simulink model "EZQStateCtrl"  (R2018b)
settings: Solver=FixedStepDiscrete  StartTime=0.0  StopTime=10.0  FixedStep=0.01  RelTol=1e-3
libraries: StateCtrlLib x1
settings Model: Creator=sn2xws  LastModifiedBy=sn2xws
settings DataIOCC: SaveFormat=StructureWithTime
settings OptimizationCC: DefaultParameterBehavior=Inlined  EnhancedBackFolding=on  PassReuseOutputArgsAs=Individual arguments  ZeroExternalMemoryAtStartup=off  ZeroInternalMemoryAtStartup=off  OptimizeBlockOrder=speed  DifferentSizesBufferReuse=on  OptimizationCustomize=off
settings DebuggingCC: ParameterTunabilityLossMsg=error
settings ModelReferenceCC: ModelReferenceNumInstancesAllowed=Single
settings SFSimCC: MATLABDynamicMemAlloc=off
settings RTWCC: SystemTargetFile=autosar.tlc  GenCodeOnly=on  TemplateMakefile=ert_default_tmf  Description=AUTOSAR  GenerateReport=on  IncludeHyperlinkInReport=on  LaunchReport=on  GenerateTraceInfo=on  GenerateTraceReport=on  GenerateTraceReportSl=on  GenerateTraceReportSf=on  GenerateTraceReportEml=on
settings CodeAppCC: ForceParamTrailComments=on  IgnoreCustomStorageClasses=off  OperatorAnnotations=on  SimulinkDataObjDesc=on  SFDataObjDesc=on  InsertBlockDesc=on
settings STFCustomTargetCC: TargetLangStandard=C99 (ISO)  MultiwordLength=256  ParMdlRefBuildCompliant=on  CompOptLevelCompliant=on  IncludeMdlTerminateFcn=off  CombineOutputUpdateFcns=on  SuppressErrorStatus=on  ERTCustomFileBanners=on  SupportNonFinite=off  SupportComplex=off  SupportContinuousTime=off  SupportNonInlinedSFcns=off  RemoveResetFunc=on  MATLABClassNameForMDSCustomization=Simulink.SoftwareTarget.ERTCustomization  AutosarCompliant=on  UseToolchainInfoCompliant=on  LookupTableObjectStructAxisOrder=2,1,3,4,...  LUTObjectStructOrderEvenSpacing=Size,Table,Breakpoints  SystemTargetFile=autosar.tlc
settings ERTTargetCC: TargetLangStandard=C99 (ISO)  ConcurrentExecutionCompliant=off  IncludeMdlTerminateFcn=off  SuppressErrorStatus=on  SupportNonFinite=off  SupportComplex=off  ModelStepFunctionPrototypeControlCompliant=off  CPPClassGenCompliant=off  AutosarCompliant=on  LookupTableObjectStructAxisOrder=2,1,3,4,...  LUTObjectStructOrderEvenSpacing=Size,Table,Breakpoints  InlinedParameterPlacement=NonHierarchical  ERTCustomFileTemplate=example_file_process.tlc

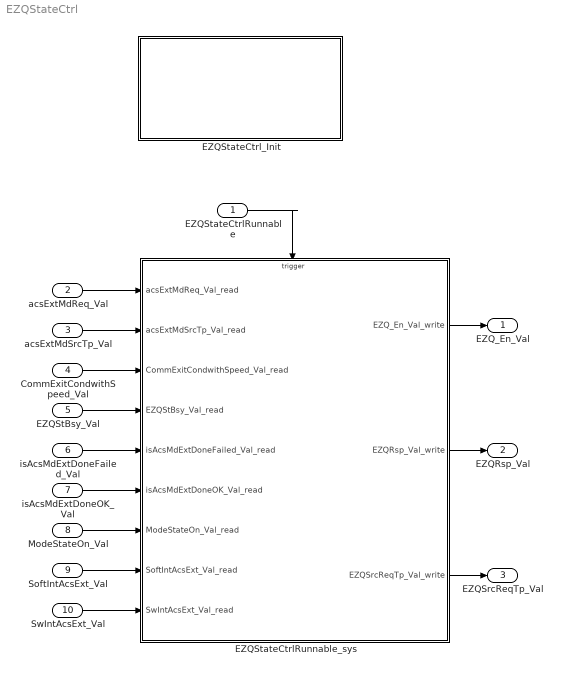
== system EZQStateCtrl ==
  EZQStateCtrlRunnable : Inport  SampleTime=0.01  OutputFunctionCall=on
  acsExtMdReq_Val : Inport  Port=2  OutDataTypeStr=boolean  PortDimensions=1
  acsExtMdSrcTp_Val : Inport  Port=3  OutDataTypeStr=Enum: SrcReqTp1  PortDimensions=1
  CommExitCondwithSpeed_Val : Inport  Port=4  OutDataTypeStr=boolean  PortDimensions=1
  EZQStBsy_Val : Inport  Port=5  OutDataTypeStr=boolean  PortDimensions=1
  isAcsMdExtDoneFailed_Val : Inport  Port=6  OutDataTypeStr=boolean  PortDimensions=1
  isAcsMdExtDoneOK_Val : Inport  Port=7  OutDataTypeStr=boolean  PortDimensions=1
  ModeStateOn_Val : Inport  Port=8  OutDataTypeStr=boolean  PortDimensions=1
  SoftIntAcsExt_Val : Inport  Port=9  OutDataTypeStr=IntEnable  PortDimensions=1
  SwIntAcsExt_Val : Inport  Port=10  OutDataTypeStr=IntEnable  PortDimensions=1
  EZQStateCtrlRunnable_sys : Subsystem
  EZQStateCtrl_Init : Subsystem
  EZQ_En_Val : Outport  OutDataTypeStr=boolean  PortDimensions=1
  EZQRsp_Val : Outport  Port=2  OutDataTypeStr=Enum: MdRspLocal1  PortDimensions=1
  EZQSrcReqTp_Val : Outport  Port=3  OutDataTypeStr=Enum: SrcReqTp1  PortDimensions=1
  wires:
  acsExtMdReq_Val/1 -> EZQStateCtrlRunnable_sys/1(acsExtMdReq_Val_read)
  acsExtMdSrcTp_Val/1 -> EZQStateCtrlRunnable_sys/2(acsExtMdSrcTp_Val_read)
  CommExitCondwithSpeed_Val/1 -> EZQStateCtrlRunnable_sys/3(CommExitCondwithSpeed_Val_read)
  EZQStBsy_Val/1 -> EZQStateCtrlRunnable_sys/4(EZQStBsy_Val_read)
  isAcsMdExtDoneFailed_Val/1 -> EZQStateCtrlRunnable_sys/5(isAcsMdExtDoneFailed_Val_read)
  isAcsMdExtDoneOK_Val/1 -> EZQStateCtrlRunnable_sys/6(isAcsMdExtDoneOK_Val_read)
  ModeStateOn_Val/1 -> EZQStateCtrlRunnable_sys/7(ModeStateOn_Val_read)
  SoftIntAcsExt_Val/1 -> EZQStateCtrlRunnable_sys/8(SoftIntAcsExt_Val_read)
  SwIntAcsExt_Val/1 -> EZQStateCtrlRunnable_sys/9(SwIntAcsExt_Val_read)
  EZQStateCtrlRunnable_sys/1(EZQ_En_Val_write) -> EZQ_En_Val/1
  EZQStateCtrlRunnable_sys/2(EZQRsp_Val_write) -> EZQRsp_Val/1
  EZQStateCtrlRunnable_sys/3(EZQSrcReqTp_Val_write) -> EZQSrcReqTp_Val/1
  EZQStateCtrlRunnable/1 -> EZQStateCtrlRunnable_sys/Trigger

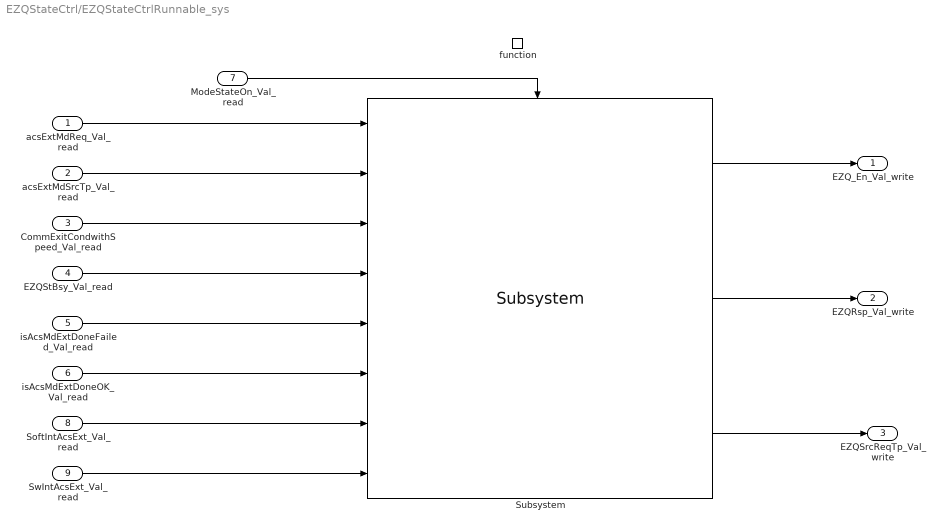
== system EZQStateCtrl/EZQStateCtrlRunnable_sys ==
  acsExtMdReq_Val_read : Inport
  acsExtMdSrcTp_Val_read : Inport  Port=2
  CommExitCondwithSpeed_Val_read : Inport  Port=3
  EZQStBsy_Val_read : Inport  Port=4
  isAcsMdExtDoneFailed_Val_read : Inport  Port=5
  isAcsMdExtDoneOK_Val_read : Inport  Port=6
  ModeStateOn_Val_read : Inport  Port=7
  SoftIntAcsExt_Val_read : Inport  Port=8  OutDataTypeStr=IntEnable
  SwIntAcsExt_Val_read : Inport  Port=9  OutDataTypeStr=IntEnable
  function : TriggerPort  TriggerType=function-call  VariantControl=(inherit)  SampleTimeType=periodic  SampleTime=-1
  Subsystem : StateCtrlLib/Subsystem  SystemSampleTime=-1
  EZQ_En_Val_write : Outport
      settings: EnsureOutportIsVirtual=on
  EZQRsp_Val_write : Outport  Port=2
      settings: EnsureOutportIsVirtual=on
  EZQSrcReqTp_Val_write : Outport  Port=3
      settings: EnsureOutportIsVirtual=on
  wires:
  ModeStateOn_Val_read/1 -> Subsystem/Enable
  acsExtMdReq_Val_read/1 -> Subsystem/1
  acsExtMdSrcTp_Val_read/1 -> Subsystem/2
  CommExitCondwithSpeed_Val_read/1 -> Subsystem/3
  SoftIntAcsExt_Val_read/1 -> Subsystem/7
  EZQStBsy_Val_read/1 -> Subsystem/4
  isAcsMdExtDoneFailed_Val_read/1 -> Subsystem/5
  SwIntAcsExt_Val_read/1 -> Subsystem/8
  isAcsMdExtDoneOK_Val_read/1 -> Subsystem/6
  Subsystem/1 -> EZQ_En_Val_write/1
  Subsystem/2 -> EZQRsp_Val_write/1
  Subsystem/3 -> EZQSrcReqTp_Val_write/1

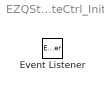
== system EZQStateCtrl/EZQStateCtrl_Init ==
  Event Listener : EventListener  EventName=reset
